simulink model "conv5x5_video_testbench"  (Simulink 7.6)
settings: Solver=FixedStepDiscrete  SolverMode=SingleTasking  StartTime=0.0  StopTime=Inf  RelTol=1e-3
PreLoadFcn:
  | xlrequire('PreLoadFcn')
undefined symbols (not defined in the file or in its folder): gray
libraries: xbsIndex_r4 x5, dspsnks4 x2, simulink x2, xbsCopyrightNotice_r4 x1
CloseFcn:
  | clear img
settings Model: Creator=alexc  LastModifiedBy=douangp
settings DataIOCC: LimitDataPoints=off  SaveOutput=off  SaveTime=off  SignalLoggingName=sigsOut
settings OptimizationCC: InitFltsAndDblsToZero=on
settings DebuggingCC: SaveWithParameterizedLinksMsg=none  SignalResolutionControl=TryResolveAllWithWarning  SolverPrmCheckMsg=none  MultiTaskDSMMsg=warning  MultiTaskCondExecSysMsg=none  StrictBusMsg=None
settings HardwareCC: TargetUnknown=on
settings RTWCC: IncludeERTFirstTime=on
settings GRTTargetCC: TargetFcnLib=ansi_tfl_tmw.mat

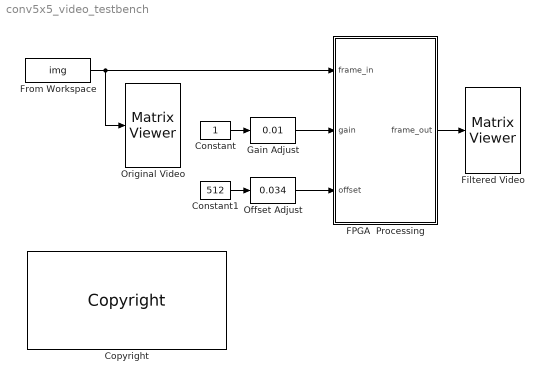
== system conv5x5_video_testbench ==
  Constant : Constant
  Constant1 : Constant  Value=512
  Copyright : xbsCopyrightNotice_r4/Copyright  copyrighttext="Copyright (c) 2011  by  Xilinx, Inc. All rights reserved.<br><br>This file contains proprietary, confidential information of Xilinx, Inc., is distributed under license from Xilinx, Inc., and may be used, copied and/or disclosed only pursuant to the terms of a valid license agreement with Xilinx, Inc. Xilinx hereby grants you a license to use this file solely for design, simulation, implementation and creation of design files limited to Xilinx devices or technologies. Use with non-Xilinx devices or technologies is expressly prohibited and immediately terminates your license unless covered by a separate agreement.<br><br>Xilinx is providing this design, code, or information \"as-is\" solely for use in developing programs and solutions for Xilinx devices, with no obligation on the part of Xilinx to provide support. By providing this design, code, or information as one possible implementation of this feature, application or standard, Xilinx is making no representation that this implementation is free from any claims of infringement. You are responsible for obtaining any rights you may require for your implementation. Xilinx expressly disclaims any warranty whatsoever with respect to the adequacy of the implementation, including but not limited to any warranties or representations that this implementation is free from claims of infringement, implied warranties of merchantability or fitness for a particular purpose.<br><br>Xilinx products are not intended for use in life support appliances, devices, or systems. Use in such applications is expressly prohibited.<br><br>Any modifications that are made to the Source Code are done at the user's sole risk and will be unsupported.<br><br>This copyright and support notice must be retained as part of this text at all times. (c) Copyright 1995-2011 Xilinx, Inc. All rights reserved."  block_type=copyright
  FPGA  Processing : Subsystem
  Filtered Video : dspsnks4/Matrix Viewer  DialogController=dspdialog.MatrixViewer  DialogControllerArgs=DataTag1  ImageParams=on  CMapStr=gray(256)  AxisColorbar=off  AxisParams=off  AxisOrigin=Upper left corner  XLabel=X-axis  YLabel=Y-axis  ZLabel=Z-axis  FigPos=[330 378 329 248]  AxisZoom=on
      settings: YMin=0  YMax=255
  From Workspace : FromWorkspace  VariableName=img  SampleTime=1  Interpolate=off  OutputAfterFinalValue=Cyclic repetition
  Gain Adjust : simulink/Math Operations/Slider Gain  SystemSampleTime=-1  low=0  gain=0.01  high=2
  Offset Adjust : simulink/Math Operations/Slider Gain  SystemSampleTime=-1  low=0  gain=0.034  high=2
  Original Video : dspsnks4/Matrix Viewer  DialogController=dspdialog.MatrixViewer  DialogControllerArgs=DataTag2  ImageParams=on  CMapStr=gray(256)  AxisColorbar=off  AxisParams=off  AxisOrigin=Upper left corner  XLabel=X-axis  YLabel=Y-axis  ZLabel=Z-axis  FigPos=[18 381 304 245]  AxisZoom=on
      settings: YMin=0  YMax=255
  wires:
  From Workspace/1 -> Original Video/1, FPGA  Processing/1(frame_in)
  FPGA  Processing/1(frame_out) -> Filtered Video/1
  Constant/1 -> Gain Adjust/1
  Gain Adjust/1 -> FPGA  Processing/2(gain)
  Constant1/1 -> Offset Adjust/1
  Offset Adjust/1 -> FPGA  Processing/3(offset)

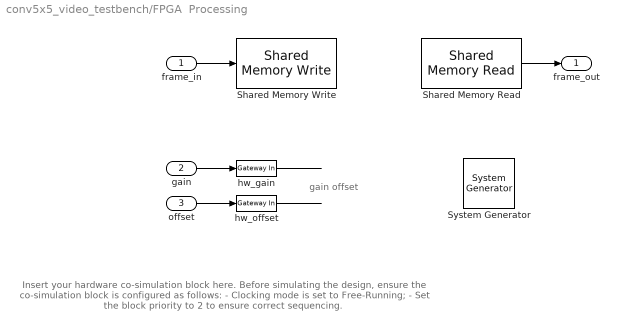
== system conv5x5_video_testbench/FPGA  Processing ==
  note: Insert your hardware co-simulation block here.  Before
      | simulating the design, ensure the co-simulation block
      | is configured as follows:
      |
      | - Clocking mode is set to Free-Running;
      | - Set the block priority to 2 to ensure correct sequencing.
  note: gain
      |
      |
      | offset
  frame_in : Inport
  gain : Inport  Port=2
  offset : Inport  Port=3
  " System Generator" : xbsIndex_r4/ System Generator  Tag=genX  SystemSampleTime=-1  xilinxfamily=kintex7  part=xc7k325t  speed=-2  package=ffg900  synthesis_tool=XST  clock_wrapper=Clock Enables  directory=./netlist  proj_type=Project Navigator  testbench=off  simulink_period=1  sysclk_period=20  dcm_input_clock_period=100  incr_netlist=off  trim_vbits=Everywhere in SubSystem  dbl_ovrd=According to Block Masks  core_generation=According to Block Masks  run_coregen=off  deprecated_control=off  eval_field=0  block_type=sysgen
  Shared Memory Read : xbsIndex_r4/Shared Memory Read  Priority=3  shmem_name='Bar'  shmem_type=Lockable memory  sample_time=1  dataType=uint8  outDims=[128 128]  isFrame=off  shmem_word=8  shmem_depth=16384  block_type=fromshmem
      settings: infoedit=Reads sequentially from a shared memory block.  block_version=VER_STRING_GOES_HERE
  Shared Memory Write : xbsIndex_r4/Shared Memory Write  Priority=1  shmem_name='Foo'  shmem_type=Lockable memory  skip_check=off  shmem_word=8  shmem_depth=16384  block_type=toshmem
      settings: infoedit=Writes scalar, vector, matrix, or frame data into a shared memory.  block_version=VER_STRING_GOES_HERE
  hw_gain : xbsIndex_r4/Gateway In  gui_display_data_type=Fixed-point  arith_type="Signed  (2's comp)"  n_bits=20  bin_pt=17  preci_type=Single  exp_width=8  frac_width=24  quantization="Round  (unbiased: +/- Inf)"  overflow=Saturate  period=1  dbl_ovrd=off  timing_constraint=None  locs_specified=off  LOCs={}  hdl_port=on  block_type=gatewayin
      settings: infoedit="Gateway in block.  Converts inputs of type Simulink integer, double and fixed point to  Xilinx fixed point type.<P><P>Hardware notes:  In hardware these blocks become top level input ports."  xl_area=[0, 0, 0, 0, 0, 0, 0]  block_version=VER_STRING_GOES_HERE
  hw_offset : xbsIndex_r4/Gateway In  gui_display_data_type=Fixed-point  arith_type=Unsigned  n_bits=10  bin_pt=0  preci_type=Single  exp_width=8  frac_width=24  quantization="Round  (unbiased: +/- Inf)"  overflow=Saturate  period=1  dbl_ovrd=off  timing_constraint=None  locs_specified=off  LOCs={}  hdl_port=on  block_type=gatewayin
      settings: infoedit="Gateway in block.  Converts inputs of type Simulink integer, double and fixed point to  Xilinx fixed point type.<P><P>Hardware notes:  In hardware these blocks become top level input ports."  xl_area=[0, 0, 0, 0, 0, 0, 0]  block_version=VER_STRING_GOES_HERE
  frame_out : Outport
  wires:
  frame_in/1 -> Shared Memory Write/1
  Shared Memory Read/1 -> frame_out/1
  gain/1 -> hw_gain/1
  offset/1 -> hw_offset/1
  hw_offset/1 -> ?
  hw_gain/1 -> ?
